simulink model "Q3_b_15"  (R2015b)
settings: Solver=VariableStepAuto  SolverMode=SingleTasking  StartTime=0.0  StopTime=1  RelTol=1e-8  AbsTol=1e-8
undefined symbols (not defined in the file or in its folder): K2
libraries: cstblocks x8
settings Model: Creator=User  LastModifiedBy=User
settings DataIOCC: LimitDataPoints=off
settings DebuggingCC: AllowSymbolicDim=on  SFUnexpectedBacktrackingDiag=error  SFNoUnconditionalDefaultTransitionDiag=error
settings ModelReferenceCC: PropagateSignalLabelsOutOfModel=on
settings GRTTargetCC: TargetLangStandard=C99 (ISO)
settings ConfigComp: CovMetricSettings=dwe  CovHtmlReporting=off  CovSaveCumulativeToWorkspaceVar=off  CovSaveSingleToWorkspaceVar=off  CovModelRefEnable=Off  CovExternalEMLEnable=on

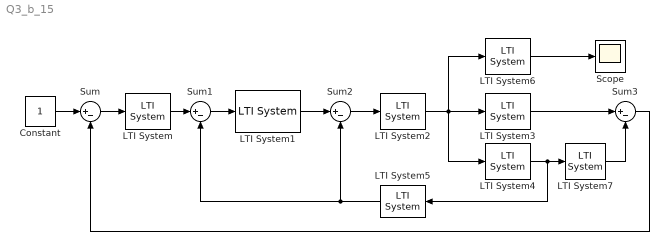
== system Q3_b_15 ==
  Constant : Constant
  LTI System : cstblocks/LTI System  sys=K3  IC=[]
  LTI System1 : cstblocks/LTI System  sys=K2*tf(1,[1 0])  IC=[]
  LTI System2 : cstblocks/LTI System  sys=K1  IC=[]
  LTI System3 : cstblocks/LTI System  sys=Pa_m  IC=[]
  LTI System4 : cstblocks/LTI System  sys=Pq  IC=[]
  LTI System5 : cstblocks/LTI System  sys=H  IC=[]
  LTI System6 : cstblocks/LTI System  sys=Pa  IC=[]
  LTI System7 : cstblocks/LTI System  sys=F  IC=[]
  Scope : Scope
  Sum{,1..3} (4 alike) : Sum  Inputs=|+-
  wires:
  Sum/1 -> LTI System/1
  Constant/1 -> Sum/1
  LTI System/1 -> Sum1/1
  Sum1/1 -> LTI System1/1
  LTI System1/1 -> Sum2/1
  Sum2/1 -> LTI System2/1
  LTI System2/1 -> LTI System6/1, LTI System3/1, LTI System4/1
  LTI System4/1 -> LTI System7/1, LTI System5/1
  LTI System5/1 -> Sum1/2, Sum2/2
  LTI System6/1 -> Scope/1
  LTI System3/1 -> Sum3/1
  LTI System7/1 -> Sum3/2
  Sum3/1 -> Sum/2
